simulink model "simident"  (Simulink 5.0)
settings: Solver=VariableStepDiscrete  SolverMode=SingleTasking  StartTime=0.0  StopTime=200  MaxStep=1e-2  RelTol=1e-3  AbsTol=1e-6
libraries: slident x1, simulink x1
settings Model: Creator=greg  LastModifiedBy=rsingh  ExtModeMexFile=ext_comm.c  ExtModeTrigMode=oneshot  ExtModeArmWhenConnect=off  ExternalInput=[]  InitialState=[]  SaveTime=off  SaveOutput=off  LimitDataPoints=off  IntegerOverflowMsg=none  BlockReductionOpt=off  BooleanDataType=off  RTWTemplateMakefile=grt_unix.tmf

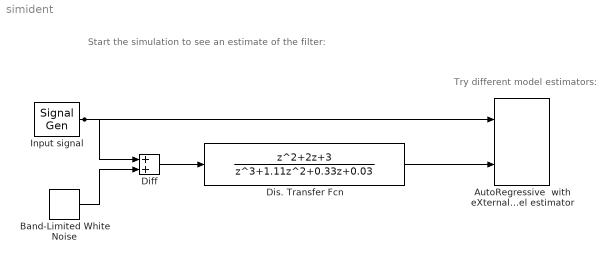
== system simident ==
  note: Try different model
      | estimators:
  note: Start the simulation to see an estimate of the filter:
  AutoRegressive  with eXternal input model estimator : slident/AutoRegressive  with eXternal input model estimator  AncestorBlock=|  order=[2 2 1]  HowOften=25  tso=0.05  npts=200  cbsim=Simulation
      | slident2/AutoRegressive 
      | with eXternal input
      | model estimator
  Band-Limited White Noise : simulink/Sources/Band-Limited White Noise  Cov=[0.001]  Ts=2*pi  seed=[23341]
  Diff : Sum  SaturateOnIntegerOverflow=on  InputSameDT=on
  Dis. Transfer Fcn : DiscreteTransferFcn  Numerator=[1 2 3]  Denominator=[1 1.11 0.33 0.03]  SampleTime=0.05
  Input signal : SignalGenerator  WaveForm=square  Amplitude=1.000000  Frequency=0.875000  Units=rad/sec
  wires:
  Diff/1 -> Dis. Transfer Fcn/1
  Dis. Transfer Fcn/1 -> AutoRegressive  with eXternal input model estimator/2
  Input signal/1 -> Diff/1, AutoRegressive  with eXternal input model estimator/1
  Band-Limited White Noise/1 -> Diff/2
